simulink model "IdentifyParameters"  (R2016b)
settings: Solver=VariableStepAuto  StartTime=0.0  StopTime=10.0  RelTol=1e-3
settings Model: DataDictionary=DataDictionary.sldd  Creator=lucadelaat  LastModifiedBy=Taeke

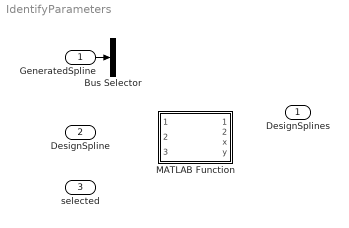
== system IdentifyParameters ==
  GeneratedSpline : Inport  OutDataTypeStr=Bus: generatedSplines  BusOutputAsStruct=on
  DesignSpline : Inport  Port=2  OutDataTypeStr=Bus: designSplineTotal  BusOutputAsStruct=on
  selected : Inport  Port=3  OutDataTypeStr=Bus: designSplineTotal  BusOutputAsStruct=on
  Bus Selector : BusSelector  OutputSignals=signal1,signal2
  MATLAB Function : MATLAB Function  TreatAsAtomicUnit=on
  DesignSplines : Outport  OutDataTypeStr=Bus: designSplineTotal
  wires:
  GeneratedSpline/1 -> Bus Selector/1

== matlab function IdentifyParameters/MATLAB Function ==
  data: angleKnee output; angleHip output; x output; designSpline input; y output; generatedSpline input; selected input
function [angleKnee, angleHip, x, y] = fcn(designSpline, generatedSpline, selected)
switch selected
case [1, 1, 0, 0]
    angleHip = designSpline.designSpline1;
    angleKnee = designSpline.designSpline2;
    x = generatedSpline.generatedSpline1;
    y = generatedSpline.generatedSpline2;
end
end
